simulink model "pseudo_integrateur"  (R2020b)
settings: Solver=VariableStepAuto  StartTime=0.0  StopTime=10.0  RelTol=1e-3
settings Model: Creator=farid  LastModifiedBy=farid

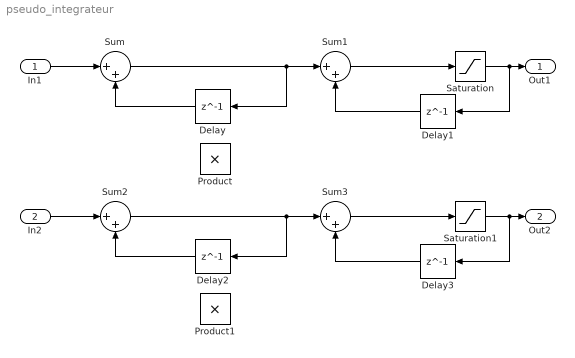
== system pseudo_integrateur ==
  In1 : Inport
  In2 : Inport  Port=2
  Delay{,1..3} (4 alike) : Delay  DelayLength=1  InitialCondition=0
  Product : Product
  Product1 : Product
  Saturation : Saturate
  Saturation1 : Saturate
  Sum{,1..3} (4 alike) : Sum  Inputs=|++
  Out1 : Outport  VectorParamsAs1DForOutWhenUnconnected=off
  Out2 : Outport  Port=2  VectorParamsAs1DForOutWhenUnconnected=off
  wires:
  In1/1 -> Sum/1
  Sum/1 -> Delay/1, Sum1/1
  Delay/1 -> Sum/2
  Delay1/1 -> Sum1/2
  Sum1/1 -> Saturation/1
  Saturation/1 -> Out1/1, Delay1/1
  Delay2/1 -> Sum2/2
  In2/1 -> Sum2/1
  Delay3/1 -> Sum3/2
  Sum3/1 -> Saturation1/1
  Saturation1/1 -> Out2/1, Delay3/1
  Sum2/1 -> Delay2/1, Sum3/1
